simulink model "Fig239"  (R2014b)
settings: Solver=ode3  StartTime=0.0  StopTime=10.007  FixedStep=2e-5  RelTol=1e-5
libraries: commutil2 x2, commfilt2 x1, commchan3 x1, commsink2 x1, commrandsrc2 x1
settings Model: Creator=Dennis Silage  LastModifiedBy=Silage
settings DataIOCC: SignalLoggingSaveFormat=ModelDataLogs
settings OptimizationCC: ExpressionDepthLimit=2147483647  InitFltsAndDblsToZero=on
settings DebuggingCC: UnderspecifiedInitializationDetection=Classic  MergeDetectMultiDrivingBlocksExec=none  SolverPrmCheckMsg=none  FcnCallInpInsideContextMsg=UseLocalSettings  StateNameClashWarn=warning
settings GRTTargetCC: CombineOutputUpdateFcns=off  GRTInterface=on

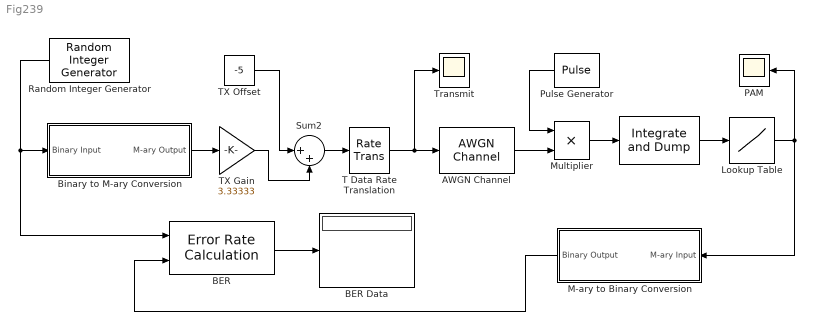
== system Fig239 ==
  " " : commfilt2/Integrate and Dump  obssamples=100  offsetsamples=0  nodump=off  roundingMode=Floor  overflowMode=off
  AWGN Channel : commchan3/AWGN Channel  InputProcessing=Inherited (this choice will be removed - see release notes)  seed=randseed  noiseMode="Signal to noise ratio  (Eb/No)"  EbNodB=40  EsNodB=20  SNRdB=10  bitsPerSym=2  Ps=13.89  Tsym=2e-3  variance=0
  BER : commsink2/Error Rate Calculation  N=8  st_delay=0  cp_mode=Entire frame  subframe=[]  PMode=Port  WsName=ErrorVec  RsMode2=off  stop=off  numErr=100  maxBits=1e6
  BER Data : Display
  Binary to M-ary Conversion : Subsystem
  Lookup Table : Lookup_n-D  NumberOfTableDimensions=1  BreakpointsForDimension1=[-2500, -833.333, 833.333, 2500]  Table=[0, 1, 2, 3]  InterpMethod=Nearest  InternalRulePriority=Speed  OutDataTypeStr=Inherit: Inherit from 'Table data'  RndMeth=Nearest  InputSameDT=on
  M-ary to Binary Conversion : Subsystem
  Multiplier : Product  RndMeth=Zero
  PAM : Scope
      settings: TimeRange=0.05  YMin=-8  YMax=8
  Pulse Generator : DiscretePulseGenerator  Amplitude=5  Period=100  PulseWidth=99  SampleTime=2e-5
  Random Integer Generator : commrandsrc2/Random Integer Generator  mul=2  seed=randseed  Ts=1e-3  frameBased=off  sampPerFrame=1  orient=off  outDataType=double
  Sum2 : Sum  Inputs=|++
  T Data Rate Translation : RateTransition  OutPortSampleTime=2e-5
  TX Gain : Gain  Gain=3.33333
  TX Offset : Constant  Value=-5
  Transmit : Scope
      settings: TimeRange=0.05  YMin=-8  YMax=8
  wires:
  BER/1 -> BER Data/1
  Lookup Table/1 -> M-ary to Binary Conversion/1(M-ary Input), PAM/1
  Multiplier/1 -> " "/1
  AWGN Channel/1 -> Multiplier/2
  Pulse Generator/1 -> Multiplier/1
  " "/1 -> Lookup Table/1
  T Data Rate Translation/1 -> AWGN Channel/1, Transmit/1
  Random Integer Generator/1 -> Binary to M-ary Conversion/1(Binary Input), BER/1
  TX Gain/1 -> Sum2/2
  Sum2/1 -> T Data Rate Translation/1
  TX Offset/1 -> Sum2/1
  Binary to M-ary Conversion/1("M-ary Output ") -> TX Gain/1
  M-ary to Binary Conversion/1(Binary Output) -> BER/2

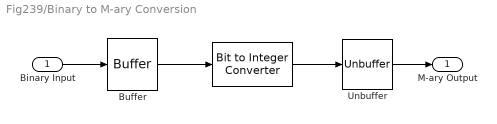
== system Fig239/Binary to M-ary Conversion ==
  Binary Input : Inport
  " " : commutil2/Bit to Integer Converter  nbits=2  bitOrder=MSB first  signedOutputValues=Unsigned  outDtype=Inherit via internal rule  outDtypeSigned=Inherit via internal rule
  Buffer : Buffer  N=2  TreatMby1Signals=One channel
  Unbuffer : Unbuffer  SampleBasedProcessing=Same as frame based
  "M-ary Output " : Outport
  wires:
  Binary Input/1 -> Buffer/1
  Buffer/1 -> " "/1
  " "/1 -> Unbuffer/1
  Unbuffer/1 -> "M-ary Output "/1

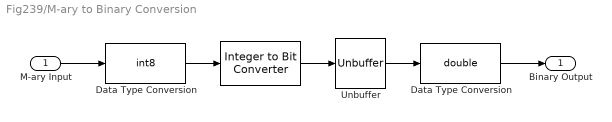
== system Fig239/M-ary to Binary Conversion ==
  M-ary Input : Inport
  " " : commutil2/Integer to Bit Converter  nbits=2  signedInputValues=Unsigned  bitOrder=MSB first  outDtype=double
  Data Type Conversion : DataTypeConversion  OutDataTypeStr=int8  RndMeth=Nearest
  "Data Type Conversion " : DataTypeConversion  OutDataTypeStr=double  RndMeth=Nearest
  Unbuffer : Unbuffer  SampleBasedProcessing=Same as frame based
  Binary Output : Outport
  wires:
  " "/1 -> Unbuffer/1
  M-ary Input/1 -> Data Type Conversion/1
  Data Type Conversion/1 -> " "/1
  Unbuffer/1 -> "Data Type Conversion "/1
  "Data Type Conversion "/1 -> Binary Output/1
